simulink model "HFCUC_unito_v1_no_sim_err_ref"  (R2021b)
settings: Solver=ode1  StartTime=0  StopTime=30  FixedStep=10e-4  MaxStep=1e-4  RelTol=10e-4  AbsTol=1e-3
InitFcn:
  | L_ind=4*10^-3;
  | alpha_hfc=10
  | alpha_ser=3
  | R_ar=1
  | init_integratore=0.001
  | delay=0.000001
settings Model: Creator=Omar  LastModifiedBy=Omar
settings DebuggingCC: UnderSpecifiedDimensionMsg=warning

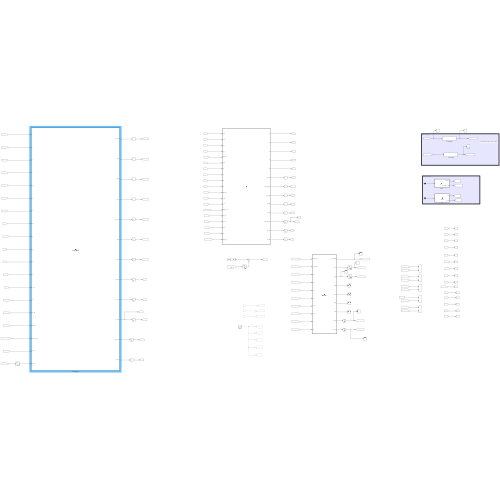
[thumbnail: Simulink's stored preview of the top-level diagram]
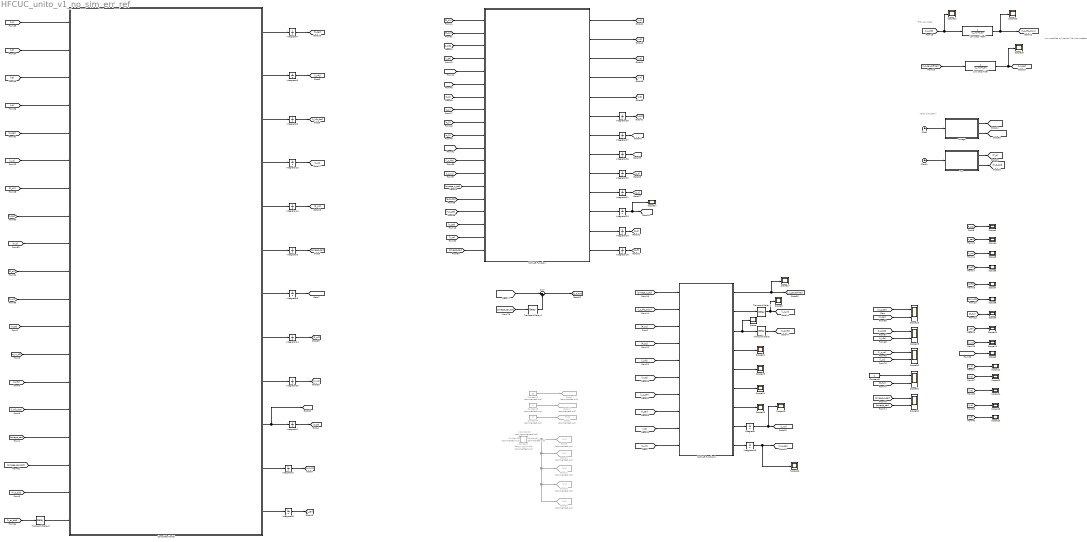
== system HFCUC_unito_v1_no_sim_err_ref ==
  note: Filtri Low Pass
  note: Valori simulativi
  note: non specifica sul paper il tau da mettere
  Clock : Clock
  Clock1 : Clock
  Complete Model : MATLAB Function  TreatAsAtomicUnit=on
  Constant : Constant  Commented=on  Value=0
  Constant1 : Subsystem  Commented=on
  Constant2 : Constant  Commented=on  Value=10
  Constant3 : Constant  Commented=on  Value=0
  Constant4 : Constant  Commented=on  Value=0
  Constant5 : Subsystem  Commented=on
  Constant6 : Subsystem  Commented=on
  Constant7 : Subsystem  Commented=on
  Constant8 : Subsystem  Commented=on
  Constant9 : Constant
  Goto1 : Goto  Commented=on  GotoTag=omega_c_ser
  Goto10 : Goto  Commented=on  GotoTag=v2
  Goto11 : Goto  Commented=on  GotoTag=v3
  Goto17 : Goto  Commented=on  GotoTag=omega_c_ser_dot
  Goto2 : Goto  Commented=on  GotoTag=T_d
  Goto26 : Goto  Commented=on  GotoTag=v4
  Goto29 : Goto  Commented=on  GotoTag=v5
  Goto9 : Goto  Commented=on  GotoTag=v1
  Integrator{,1..3,5..6,8..10,13,18..22,25..28} (19 alike) : Integrator
  Integrator14 : Integrator  InitialCondition=init_integratore
  Integrator24 : Integrator  InitialCondition=init_integratore
  Integrator7 : Integrator  InitialCondition=init_integratore
  Low pass filter : TransferFcn  Denominator=[L_ind R_ar]
  Low pass filter1 : TransferFcn  Denominator=[L_ind R_ar]
  MATLAB Function : MATLAB Function  TreatAsAtomicUnit=on
  MATLAB Function2 : MATLAB Function  TreatAsAtomicUnit=on
  Omega : MATLAB Function  TreatAsAtomicUnit=on
  Scope{,1..27} (28 alike) : Scope
  Scope{28..32} (5 alike) : Scope  NumInputPorts=2
  Sum : Sum  Inputs=|-+
  TD : MATLAB Function  TreatAsAtomicUnit=on
  Transport Delay{,1..3} (4 alike) : TransportDelay  DelayTime=delay
  wires:
  Clock/1 -> Omega/1(t)
  TD/1(T_d) -> [T_d]
  Clock1/1 -> TD/1(t)
  Omega/1(omega_c) -> [omega_c_ser]
  [i_c_hfc] -> Scope21/1, Low pass filter1/1
  Low pass filter1/1 -> Scope20/1, [i_c_hfc_slow]
  [i_c_ser_tofilter] -> Low pass filter/1
  Constant/1 -> Goto29/1, Goto26/1, Goto11/1, Goto10/1, Goto9/1
  [P_o2] -> Scope1/1
  Omega/2(omega_c_dot) -> [omega_c_ser_dot]
  Constant2/1 -> Goto1/1
  [V_ser] -> Scope4/1
  [V_uc] -> Scope5/1
  [V_at] -> Scope6/1
  [i_hfc] -> Scope7/1
  [q_in_o2] -> Scope8/1
  [P_h2] -> Scope9/1
  [i_ser] -> Scope10/1
  [i_uc] -> Scope11/1
  Constant3/1 -> Goto17/1
  Constant4/1 -> Goto2/1
  [v1] -> Scope12/1
  [v2] -> Scope13/1
  [v3] -> Scope14/1
  [v4] -> Scope15/1
  [v5] -> Scope16/1
  Integrator27/1 -> [alpha_hfc]
  [omega_c_ser] -> MATLAB Function/14(omega_c_ser)
  MATLAB Function/13(z_3_dot) -> Integrator18/1
  MATLAB Function/6(I_e4_dot) -> Integrator28/1
  [alpha_hfc] -> MATLAB Function/5(alpha_hfc)
  MATLAB Function/7(alpha_hfc_dot) -> Integrator27/1
  MATLAB Function/9(z_0_dot) -> Integrator22/1
  MATLAB Function/1(v1) -> [v1]
  Integrator19/1 -> [z_2]
  MATLAB Function/5(v5) -> [v5]
  [i_c_hfc] -> MATLAB Function/12(i_c_hfc)
  Integrator21/1 -> [z_1]
  [i_c_uc] -> MATLAB Function/13(i_c_uc)
  Integrator22/1 -> [z_0]
  MATLAB Function/4(v4) -> [v4]
  MATLAB Function/12(z_2_dot) -> Integrator19/1
  Integrator26/1 -> [v41_s]
  [z_2] -> MATLAB Function/9(z_2)
  Integrator18/1 -> [z_3]
  [alpha_ser] -> MATLAB Function/11(alpha_ser)
  MATLAB Function/2(v2) -> [v2]
  [P_o2] -> MATLAB Function/2(P_o2)
  MATLAB Function/8(v41_s_dot) -> Integrator26/1
  [z_3] -> MATLAB Function/10(z_3)
  Integrator28/1 -> [I_e4]
  [P_h2] -> MATLAB Function/1(P_h2)
  [i_hfc] -> MATLAB Function/3(i_hfc)
  MATLAB Function/11(alpha_ser_dot) -> Integrator20/1
  [v41_s] -> MATLAB Function/6(v_41s)
  MATLAB Function/10(z_1_dot) -> Integrator21/1
  Integrator20/1 -> Scope27/1, [alpha_ser]
  MATLAB Function/3(v3) -> [v3]
  [z_0] -> MATLAB Function/7(z_0)
  [z_1] -> MATLAB Function/8(z_1)
  [I_e4] -> MATLAB Function/4(I_e4)
  [V_c_ser] -> MATLAB Function/16(V_c_ser)
  Complete Model/12(i_ser_dot) -> Integrator8/1
  Integrator3/1 -> [omega_ser]
  Complete Model/2(x_1_dot) -> Integrator5/1
  Integrator6/1 -> [i_hfc_dot]
  [i_hfc] -> Complete Model/14(i_hfc)
  Complete Model/3(x_2_dot) -> Integrator6/1
  Complete Model/10(V_at_dot) -> [V_at_dot], Integrator1/1
  [i_hfc_dot] -> Complete Model/15(i_hfc_dot)
  Complete Model/6(x_3_dot) -> Integrator3/1
  [v4] -> Complete Model/4(v4)
  [v1] -> Complete Model/1(v1)
  [V_at] -> Complete Model/12(V_at)
  [q_in_o2] -> Complete Model/13(q_in_o2)
  Integrator14/1 -> [P_h2]
  Integrator13/1 -> [i_uc]
  Complete Model/7(x_4_dot) -> Integrator9/1
  [i_ser] -> Complete Model/8(i_ser)
  Complete Model/9(V_uc_dot) -> Integrator25/1
  Complete Model/8(P_o2_dot) -> Integrator24/1
  [P_o2] -> Complete Model/10(P_o2)
  Complete Model/11(q_in_o2_dot) -> Integrator2/1
  Integrator8/1 -> [i_ser]
  [v3] -> Complete Model/3(v3)
  Integrator24/1 -> [P_o2]
  Integrator1/1 -> [V_at]
  Integrator25/1 -> [V_uc]
  Complete Model/4(i_uc_dot) -> Integrator13/1
  [omega_ser] -> Complete Model/16(omega_ser)
  [v2] -> Complete Model/2(v2)
  Complete Model/5(P_h2_dot) -> Integrator14/1
  [i_uc] -> Complete Model/6(i_uc)
  Integrator2/1 -> [q_in_o2]
  Complete Model/1(V_ser_dot) -> Integrator7/1
  [P_h2] -> Complete Model/7(P_h2)
  [T_d_dot] -> Complete Model/18(T_d_dot)
  [T_d] -> Complete Model/9(T_d)
  [V_ser] -> Complete Model/5(V_ser)
  [V_uc] -> Complete Model/11(V_uc)
  Integrator7/1 -> [V_ser]
  [i_c_hfc_slow] -> MATLAB Function2/2(i_c_hfc_slow)
  [omega_c_ser] -> MATLAB Function2/1(omega_c_ser)
  [v5] -> MATLAB Function2/9(v5)
  MATLAB Function2/1(i_c_ser_tofilter) -> [i_c_ser_tofilter], Scope17/1
  MATLAB Function2/3(i_c_hfc) -> Transport Delay/1, Scope/1
  [P_h2] -> MATLAB Function2/3(P_h2)
  [P_o2] -> MATLAB Function2/4(P_o2)
  [i_hfc] -> MATLAB Function2/5(i_hfc)
  [V_at] -> MATLAB Function2/6(V_at)
  [i_c_ser] -> MATLAB Function2/7(i_c_ser)
  [V_ser] -> MATLAB Function2/8(V_ser)
  MATLAB Function2/2(i_c_uc) -> Transport Delay1/1
  MATLAB Function2/4(V_thfc) -> Scope22/1
  MATLAB Function2/5(V_ohm) -> Scope23/1
  Integrator5/1 -> [i_hfc]
  Integrator9/1 -> [omega_ser_dot]
  MATLAB Function2/6(E_hfc) -> Scope24/1
  MATLAB Function2/7(V_hfc) -> Scope25/1
  Low pass filter/1 -> Scope18/1, [i_c_ser]
  [omega_c_ser_dot] -> Sum/1
  Sum/1 -> [e_5_dot]
  [omega_ser_dot] -> Transport Delay2/1
  Transport Delay2/1 -> Sum/2
  [e_5_dot] -> MATLAB Function/15(e_5_dot)
  [I_v5] -> MATLAB Function2/10(I_v5)
  MATLAB Function2/8(I_v5_dot) -> Integrator/1
  MATLAB Function2/9(V_c_ser) -> Integrator10/1
  Integrator/1 -> Scope19/1, [I_v5]
  Integrator10/1 -> Scope26/1, [V_c_ser]
  [V_ser] -> MATLAB Function/17(V_ser)
  [i_uc] -> MATLAB Function/18(i_uc)
  [omega_ser] -> MATLAB Function/19(omega_ser)
  [omega_ser_dot] -> Complete Model/17(omega_ser_dot)
  Transport Delay/1 -> [i_c_hfc]
  Transport Delay1/1 -> [i_c_uc], Scope3/1
  TD/2(T_d_dot) -> [T_d_dot]
  [V_at_dot] -> Transport Delay3/1
  Transport Delay3/1 -> Complete Model/19("V_at_dot ")
  [V_c_ser] -> Scope28/1
  [V_ser] -> Scope28/2
  [i_hfc] -> Scope29/2
  [i_c_hfc] -> Scope29/1
  [i_c_uc] -> Scope30/1
  [i_uc] -> Scope30/2
  [P_h2] -> Scope31/2
  Constant9/1 -> Scope31/1
  [omega_c_ser] -> Scope32/1
  [omega_ser] -> Scope32/2
  [omega_ser_dot] -> Scope2/1

== system HFCUC_unito_v1_no_sim_err_ref/Constant1 ==

== system HFCUC_unito_v1_no_sim_err_ref/Constant5 ==

== system HFCUC_unito_v1_no_sim_err_ref/Constant6 ==

== system HFCUC_unito_v1_no_sim_err_ref/Constant7 ==

== system HFCUC_unito_v1_no_sim_err_ref/Constant8 ==

== matlab function HFCUC_unito_v1_no_sim_err_ref/Complete Model ==
  data: v1 input; V_ser_dot output; v2 input; v3 input; v4 input; V_ser input; i_uc input; P_h2 input; i_ser input; T_d input; P_o2 input; V_uc input; V_at input; q_in_o2 input; i_hfc input; i_hfc_dot input; omega_ser input; omega_ser_dot input; T_d_dot input; x_1_dot output; x_2_dot output; i_uc_dot output; P_h2_dot output; x_3_dot output; x_4_dot output; P_o2_dot output; V_uc_dot output; V_at_dot output; q_in_o2_dot output; i_ser_dot output; V_at_dot input
function [V_ser_dot,x_1_dot,x_2_dot,i_uc_dot,P_h2_dot,x_3_dot,x_4_dot,P_o2_dot,V_uc_dot,V_at_dot,q_in_o2_dot,i_ser_dot] = CompleteModel(v1,v2,v3,v4,V_ser,i_uc,P_h2,i_ser,T_d,P_o2,V_uc,V_at,q_in_o2,i_hfc,i_hfc_dot,omega_ser,omega_ser_dot,T_d_dot,V_at_dot)
L_ind=4*10e-3;
k_b=0.1;
b=0.1;
R_ar=1;
k_m=5;
J=0.5;
n_g=0.3;
R_at=0.08;
R_ohm=0.06;
deltas_1=170;
tau_o2=6.74;
k_o2=2.52e-3;
tau_h2=3.37;
k_h2=8.48e-4;
tau_qh2=2e-2;
tau_qo2=2e-2;
C_b=14e-3; % c_b messo uguale a c_d non lo da sul paper preso da loro paper vecchio
C_d=68.5e-3; %le ho messe uguali ma manca questo parametro nel paper
T_hfc=298.15;
T_st=353;
F_0=96485.3415;
L=35e-4;
L_uc=140e-4;
R_uc=1.2e+4;
C_uc=125;
n=185;
k_gamma1=2.28027e-7;%sui parametri dice cosi 2.28027e-7 ma a pag4 dice che vale n/4*F_0
R_g=8.31417;

deltag_1=-4.4e3;
P_c_h2=1.01e5;



%supposizioni ora le ho messe le misure che ho
v1_dot=0;
%V_at_dot=0;
%T_d_dot=0;

%Definisco i_hfc=x_1 i_hfc_dot=x_2 omega_ser=x_3 omega_ser_dot=x_4

Omega1=(1/(L*C_b))*((3/2)*i_hfc-i_hfc*v1-i_ser);%C_b non lo ho come parametro
Omega2=((n*R_g*T_st)/(4*F_0*L))*(1/(tau_o2*k_o2*P_o2));
Omega3=(-1/C_b)*i_uc*(1-v1);
H1=(1/(2*C_b))*(i_hfc+i_uc-2*i_ser);
H2=(1/L)*(1/(2*C_b)*(-i_hfc+2*i_ser)+v1_dot*V_ser-i_hfc_dot-V_at_dot+(n*R_g*T_st)/(2*F_0)*((1/P_h2)*((-1/tau_h2)*P_h2+1/(tau_h2*k_h2)*(v3-2*k_gamma1*i_hfc))+1/(2*P_o2)*(-1/tau_o2*P_o2-k_gamma1/(tau_o2*k_o2)*i_hfc)));
%H2=(1/L)*((1/(2*C_b))*(-i_hfc+2*i_ser)+v1_dot*V_ser-i_hfc_dot-V_at_dot+((n*R_g*T_st)/(2*F_0))*((1/P_h2)*((-1/tau_h2)*P_h2+(1/(tau_h2*k_h2))*(v3-2*k_gamma1*i_hfc))+(1/(2*P_o2))*((-1/tau_o2)*P_o2-((k_gamma1)/(tau_o2*k_o2))*i_hfc)));
H3=(1/(2*L_uc))*(-V_ser+2*V_uc);
H4=(-1/tau_h2)*P_h2-((2*k_gamma1)/(tau_h2*k_h2))*i_hfc;
H5=(1/J)*(-((k_m*k_b)/(L_ind)-(b^2/J))*omega_ser-k_m*((b/J)+(R_ar/L_ind))*i_ser-n_g*((b/J)*T_d-T_d_dot));


V_ser_dot=H1-(1/C_b)*i_hfc*v1-(1/C_b)*i_uc*(H3*L_uc)/V_ser;


%calcolo i_hfc derivata seconda
x_1_dot=i_hfc_dot;
x_2_dot=H2+Omega1*v1+Omega3*v2+Omega2*v4;
%i_hfc_ddot=H2+Omega1*v1+Omega2*v4+Omega3*v2;



i_uc_dot=H3-(1/L_uc)*V_ser*v2;

P_h2_dot=H4+(1/(tau_h2*k_h2))*v3;

%derivata seconda omega_ser
x_3_dot=omega_ser_dot;
x_4_dot=H5+(k_m/(L_ind*J))*V_ser;
%omega_ser_ddot=H5+(k_m/(L_ind*J))*V_ser;


V_at_dot=i_hfc/C_d-(V_at/(R_at*C_d));

%Servomotor

i_ser_dot=(1/L_ind)*(-R_ar*i_ser-k_b*omega_ser+V_ser);

%PRESA DA HFC
q_in_o2_dot=(1/(tau_qo2))*(-q_in_o2+v4);
P_o2_dot=(-1/tau_o2)*P_o2+(1/(tau_o2*k_o2))*(q_in_o2-k_gamma1*i_hfc);

%Presa da uc
V_uc_dot=(-1/(R_uc*C_uc))*(V_uc+R_uc*i_uc);





end

== matlab function HFCUC_unito_v1_no_sim_err_ref/Omega ==
  data: t input; omega_c output; omega_c_dot output
function [omega_c,omega_c_dot]  = Omega(t)
omega_c=100+100*sin(0.2*t);
omega_c_dot=20*cos(0.2*t);
end

== matlab function HFCUC_unito_v1_no_sim_err_ref/TD ==
  data: t input; T_d output; T_d_dot output
function [T_d,T_d_dot] = Omega(t)
T_d=10+8*sin(0.2*t)+2*sin(10*t);
T_d_dot=1.6*cos(0.2*t) + 20*cos(10*t);
end

== matlab function HFCUC_unito_v1_no_sim_err_ref/MATLAB Function ==
  data: P_h2 input; P_o2 input; v1 output; v2 output; v3 output; v4 output; v5 output; I_e4_dot output; alpha_hfc_dot output; v41_s_dot output; z_0_dot output; z_1_dot output; alpha_ser_dot output; z_2_dot output; z_3_dot output; i_hfc input; I_e4 input; alpha_hfc input; v_41s input; z_0 input; z_1 input; z_2 input; z_3 input; alpha_ser input; i_c_hfc input; i_c_uc input; omega_c_ser input; e_5_dot input; V_c_ser input; V_ser input; i_uc input; omega_ser input
function [v1,v2,v3,v4,v5,I_e4_dot,alpha_hfc_dot,v41_s_dot,z_0_dot,z_1_dot,alpha_ser_dot,z_2_dot,z_3_dot] = fcn(P_h2,P_o2,i_hfc,I_e4,alpha_hfc,v_41s,z_0,z_1,z_2,z_3,alpha_ser,i_c_hfc,i_c_uc,omega_c_ser,e_5_dot,V_c_ser,V_ser,i_uc,omega_ser)
%% parametri modello
L_ind=4*10e-3;
k_b=0.1;
b=0.1;
R_ar=1;
k_m=5;
J=0.5;
n_g=0.3;
R_at=0.08;
R_ohm=0.06;
deltas_1=170;
tau_o2=6.74;
k_o2=2.52e-3;
tau_h2=3.37;
k_h2=8.48e-4;
tau_qh2=2e-2;
tau_qo2=2e-2;
C_b=14e-3; % c_b messo uguale a c_d non lo da sul paper preso da loro paper vecchio
C_d=68.5e-3; %le ho messe uguali ma manca questo parametro nel paper
T_hfc=298.15;
T_st=353;
F_0=96485.3415;
L=35e-4;
L_uc=140e-4;
R_uc=1.2e+4;
C_uc=125;
n=185;
k_gamma1= n/(4*F_0);%sui parametri dice cosi 2.28027e-7 ma a pag4 dice che vale n/4*F_0
R_g=8.31417;

deltag_1=-4.4e3;
P_c_h2=1;



%% parametri


alpha_min=0.7;
P_c_h2=1;
omega_h=60;
epsilon_h=0.03;
xsi_s=0.01;
gamma_1s=20;
mu=0.05;
alpha_hmin=1;
gamma_h=10;
ni_h=0.01;
mu_s=0.08;
xsi=0.01;
mu_h=0.04;
omega_1s=30;
alpha_sermin=0.7;
delta_1s=10;

%% Errori


e_1=V_c_ser-V_ser;
e_2=i_c_hfc-i_hfc;
e_3=i_c_uc-i_uc;
e_4=P_c_h2-P_h2;
e_5=omega_c_ser-omega_ser;

%% controllo v1,v2 transistor
v1=-0.5*sign(e_1);
v2=0.5*sign(e_3);

%% controllo v3 PI
k_p1=0.45;
k_i1=1.56;

I_e4_dot=e_4;

v3=k_h2*P_h2+2*k_gamma1*i_hfc+k_p1*e_4+k_i1*I_e4;


%% controllo v4

%differentiator
lambda_0=100;
lambda_1=30;
%mi da zo =e_2 e z_1=e_2_dot
z_0_dot=-lambda_1*sqrt(abs(z_0-e_2))*sign(z_0-e_2)+z_1;
z_1_dot=-lambda_0*sign(lambda_1*sqrt(abs(z_0-e_2))*sign(z_0-e_2));

c_2s=100;%scelto io non lo specifica

sigma_2s=z_1+c_2s*e_2;


if alpha_hfc>alpha_hmin
    alpha_hfc_dot=omega_h*sqrt(gamma_h/2)*sign(abs(sigma_2s)-mu_h);
else
    alpha_hfc_dot=ni_h;
end

beta_hfc=2*epsilon_h*alpha_hfc;%sul paper è h e basta il pedice di alpha

v41_s_dot=(beta_hfc/2)*sign(sigma_2s);
v4_s=alpha_hfc*sqrt(abs(sigma_2s))*sign(sigma_2s)+v_41s;


v4=((4*L*F_0*tau_o2*k_o2*P_o2)/(n*R_g*T_st))*v4_s;

%% controllo v5
%differentiator
lambda_3=120;
lambda_2=40;

c_ser1=100;%a caso non è riportato sul paper

sigma_ser=e_5_dot+c_ser1*e_5;

z_2_dot=-lambda_2*sqrt(abs(z_2-sigma_ser))*sign(z_2-sigma_ser)+z_3;
z_3_dot=-lambda_3*sign(lambda_2*sqrt(abs(z_2-sigma_ser))*sign(z_2-sigma_ser));

%Omega_S=alpha_ser^2*sigma_ser^2+gamma_1s*abs(sigma_ser)^(3/2)*sign(sigma_ser)*z_1+alpha_ser*abs(sigma_ser)*z_1^2+0.25*z_1^4;%lui ne usa una più semplice dice
Omega_S=sigma_ser^2+delta_1s*z_3^2;

if alpha_ser>=alpha_sermin
    alpha_ser_dot=omega_1s*sqrt(gamma_1s/2)*sign(Omega_S-mu_s);
else 
    alpha_ser_dot=xsi_s;
end


v5=-alpha_ser*(sign(sigma_ser)+(1/2)*sign(z_3));

% %% saturazione
% if v4>=20
%     v4=20;
% elseif v4<=-20
%     v4=-20;
% end
% if v5>=20
%     v5=20;
% elseif v5<=-20
%     v5=-20;
% end
% % if v3>=20
% %     v3=20;
% % elseif v3<=-20
% %     v3=-20;
% % end

end

== matlab function HFCUC_unito_v1_no_sim_err_ref/MATLAB Function2 ==
  data: omega_c_ser input; i_c_hfc_slow input; P_h2 input; P_o2 input; i_hfc input; V_at input; i_c_ser input; V_ser input; v5 input; i_c_ser_tofilter output; i_c_uc output; i_c_hfc output; V_thfc output; V_ohm output; E_hfc output; V_hfc output; I_v5 input; I_v5_dot output; V_c_ser output
function [i_c_ser_tofilter,i_c_uc,i_c_hfc,V_thfc,V_ohm,E_hfc,V_hfc,I_v5_dot,V_c_ser] = Reference(omega_c_ser,i_c_hfc_slow,P_h2,P_o2,i_hfc,V_at,i_c_ser ,V_ser,v5,I_v5)


L_ind=4*10e-3;
k_b=0.1;
b=0.1;
R_ar=1;
k_m=5;
J=0.5;
n_g=0.3;
R_at=0.08;
R_ohm=0.06;
deltas_1=170;
tau_o2=6.74;
k_o2=2.52e-3;
tau_h2=3.37;
k_h2=8.48e-4;
tau_qh2=2e-2;
tau_qo2=2e-2;
C_b=14e-3; % c_b messo uguale a c_d non lo da sul paper preso da loro paper vecchio
C_d=68.5e-3; %le ho messe uguali ma manca questo parametro nel paper
T_hfc=298.15;
T_st=353;
F_0=96485.3415;
L=35e-4;
L_uc=140e-4;
R_uc=1.2e+4;
C_uc=125;
n=185;
k_gamma1=2.28027e-7;%sui parametri dice cosi 2.28027e-7 ma a pag4 dice che vale n/4*F_0
R_g=8.31417;

deltag_1=-4.4e3;
P_c_h2=1.01e5;


I_v5_dot=v5;
V_c_ser=((L_ind*J)/k_m)*I_v5;

E_hfc=(deltag_1/(2*F_0))+(deltas_1/(2*F_0))*(T_st-T_hfc)+((R_g*T_st)/(2*F_0))*((log(abs(P_h2)))+1/2*log(abs(P_o2)));
V_ohm=i_hfc*R_ohm;
V_hfc=E_hfc-V_ohm-V_at;

V_thfc=185*V_hfc;
i_c_ser_tofilter=-k_b*omega_c_ser+V_c_ser;
i_c_hfc=i_c_ser*(V_c_ser/V_thfc);


i_c_uc=(V_thfc/V_ser)*(i_c_hfc-i_c_hfc_slow);


end
